simulink model "AD_SOAR_c7_V2f_c73_Clean_FullOrderControllerTest"  (R2022b)
settings: Solver=ode4  StartTime=0.0  StopTime=TMax  FixedStep=Control.DT  RelTol=1e-3
values from neighbouring files (symbols this model uses):
  dLPF_slow = c2d(ss(LPF_slow),Control.DT)    [C_BL_SOAR25_V2f_c73_Clean.m]    (also in C_BL_SOAR25_V2f_c73_Clean_original.m)
  DT = 0.0125    [hinf_controller.m]
  LPF_SetSmooth = Af_LPF(2*pi/10,1,Control.DT,1)    [C_BL_SOAR25_V2f_c73_Clean.m]    (also in C_BL_SOAR25_V2f_c73_Clean_original.m)
  OutList =     [OutList.mat]
  S_LowBPLim = 1    [C_BL_SOAR25_V2f_c73_Clean.m]    (also in C_BL_SOAR25_V2f_c73_Clean_original.m)
undefined symbols (not defined in the file or in its folder): Control, DiscIntNeverNeededParam, Downratelimiter, OLControlParams, Parameters, PitchControlParams, rpm2radps, Simulation, strmatch, TorqueControlParams, Upratelimiter
libraries: cstblocks x4, simulink x2, simulink_extras x1
settings Model: Creator=Hazim Namik  LastModifiedBy=aoifework
settings SolverCC: AlgebraicLoopSolver=LineSearch
settings DataIOCC: LimitDataPoints=on  SaveFormat=Array  ReturnWorkspaceOutputs=off  SignalLoggingName=sigsOut
settings OptimizationCC: BlockReduction=off  BooleanDataType=off  ReuseModelBlockBuffer=on  LifeSpan=inf
settings DebuggingCC: SaveWithParameterizedLinksMsg=none  UnderspecifiedInitializationDetection=Classic  MergeDetectMultiDrivingBlocksExec=none  UnconnectedInputMsg=warning  UnconnectedOutputMsg=warning  UnconnectedLineMsg=warning  AllowSymbolicDim=off  PregeneratedLibrarySubsystemCodeDiagnostic=none  SFUnexpectedBacktrackingDiag=warning  SFNoUnconditionalDefaultTransitionDiag=warning  SFExecutionAtInitializationDiag=none  ArithmeticOperatorsInVariantConditions=warning
settings HardwareCC: ProdBitPerPointer=32  ProdBitPerSizeT=32  ProdBitPerPtrDiffT=32  ProdLargestAtomicFloat=None  ProdIntDivRoundTo=Undefined  ProdEndianess=Unspecified  ProdWordSize=32  ProdHWDeviceType=32-bit Generic  TargetBitPerLong=64  TargetBitPerPointer=64  TargetBitPerSizeT=64  TargetBitPerPtrDiffT=64  TargetLongLongMode=on  TargetIntDivRoundTo=Zero  TargetEndianess=LittleEndian  TargetWordSize=64  TargetHWDeviceType=MATLAB Host  ProdEqTarget=off
settings ModelReferenceCC: EnableRefExpFcnMdlSchedulingChecks=on  PropagateSignalLabelsOutOfModel=off
settings SFSimCC: SimUseLocalCustomCode=off  CustomCodeUndefinedFunction=UseInterfaceOnly
settings RTWCC: RTWUseLocalCustomCode=off  DLArmComputeVersion=19.05
settings CodeAppCC: StateflowObjectComments=on
settings GRTTargetCC: TargetLangStandard=C89/C90 (ANSI)
settings ConfigComp: CovMetricSettings=dw  CovSaveCumulativeToWorkspaceVar=on  CovSaveSingleToWorkspaceVar=on  CovExternalEMLEnable=off  CovSFcnEnable=off

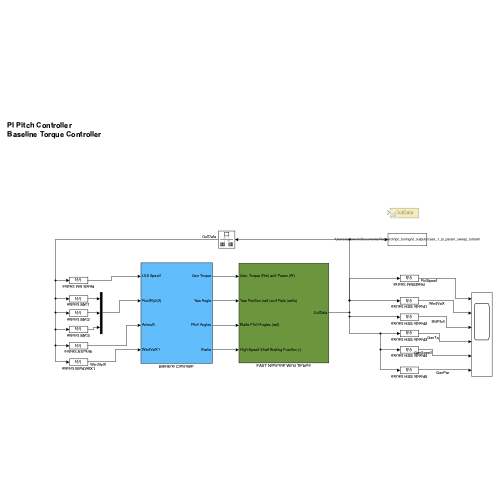
[thumbnail: Simulink's stored preview of the top-level diagram]
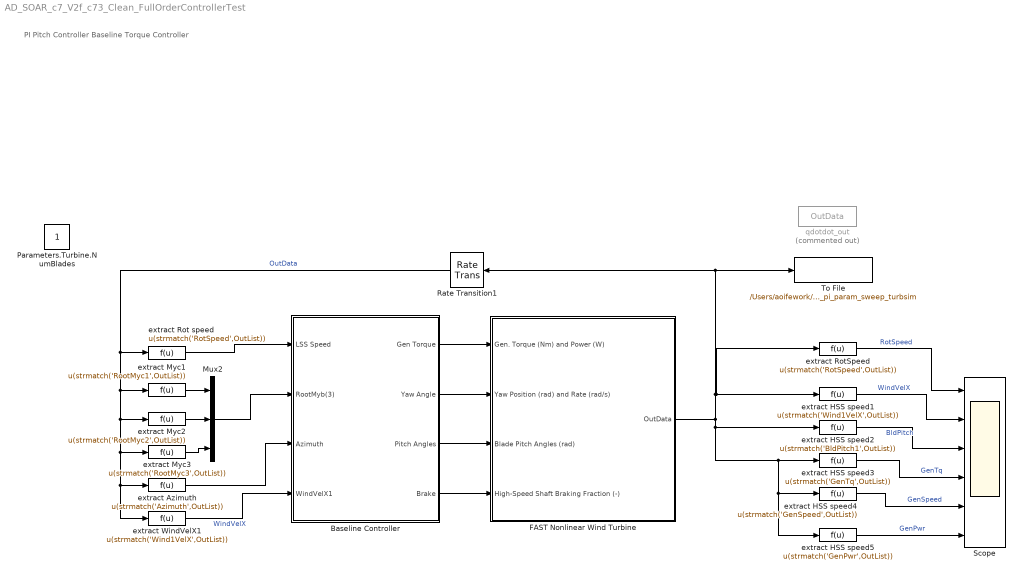
== system AD_SOAR_c7_V2f_c73_Clean_FullOrderControllerTest ==
  note: PI Pitch Controller
      | Baseline Torque Controller
  Baseline Controller : Subsystem
  FAST Nonlinear Wind Turbine : Subsystem  mask(FAST Nonlinear Wind Turbine){}
      mask help: This block contains the FAST S-Function.
      mask init:
      | clear FAST_SFunc
  Mux2 : Mux  Inputs=3
  Rate Transition1 : RateTransition
  Scope : Scope  NumInputPorts=6
  To File : ToFile  Filename=/Users/aoifework/Documents/Research/ipc_tuning/sl_outputs/case_1_pi_param_sweep_turbsim  MatrixName=OutData  SaveFormat=Timeseries
  extract Azimuth : Fcn  Expr=u(strmatch('Azimuth',OutList))
  extract HSS speed1 : Fcn  Expr=u(strmatch('Wind1VelX',OutList))
  extract HSS speed2 : Fcn  Expr=u(strmatch('BldPitch1',OutList))
  extract HSS speed3 : Fcn  Expr=u(strmatch('GenTq',OutList))
  extract HSS speed4 : Fcn  Expr=u(strmatch('GenSpeed',OutList))
  extract HSS speed5 : Fcn  Expr=u(strmatch('GenPwr',OutList))
  extract Myc1 : Fcn  Expr=u(strmatch('RootMyc1',OutList))
  extract Myc2 : Fcn  Expr=u(strmatch('RootMyc2',OutList))
  extract Myc3 : Fcn  Expr=u(strmatch('RootMyc3',OutList))
  extract Rot speed : Fcn  Expr=u(strmatch('RotSpeed',OutList))
  extract RotSpeed : Fcn  Expr=u(strmatch('RotSpeed',OutList))
  extract WindVelX1 : Fcn  Expr=u(strmatch('Wind1VelX',OutList))
  qdotdot_out : ToWorkspace  Commented=on  VariableName=OutData  SaveFormat=Structure With Time  SampleTime=-1
  Parameters.Turbine.NumBlades : Constant  IOType=siggen
  wires:
  Rate Transition1/1 -> extract Myc1/1, extract Myc2/1, extract Myc3/1, extract WindVelX1/1, extract Azimuth/1, extract Rot speed/1  "OutData"
  Baseline Controller/1(Gen Torque) -> FAST Nonlinear Wind Turbine/1(Gen. Torque (Nm) and Power (W))
  Baseline Controller/2(Yaw Angle) -> FAST Nonlinear Wind Turbine/2(Yaw Position (rad) and Rate (rad/s))
  Baseline Controller/3(Pitch Angles) -> FAST Nonlinear Wind Turbine/3(Blade Pitch Angles (rad))
  Baseline Controller/4(Brake) -> FAST Nonlinear Wind Turbine/4(High-Speed Shaft Braking Fraction (-))
  extract HSS speed1/1 -> Scope/2  "WindVelX"
  extract HSS speed2/1 -> Scope/3  "BldPitch"
  extract HSS speed3/1 -> Scope/4  "GenTq"
  extract HSS speed4/1 -> Scope/5  "GenSpeed"
  extract HSS speed5/1 -> Scope/6  "GenPwr"
  extract Rot speed/1 -> Baseline Controller/1(LSS Speed)
  FAST Nonlinear Wind Turbine/1(OutData) -> Rate Transition1/1, To File/1, extract RotSpeed/1, extract HSS speed1/1, extract HSS speed5/1, extract HSS speed4/1, extract HSS speed3/1, extract HSS speed2/1
  extract RotSpeed/1 -> Scope/1  "RotSpeed"
  extract Myc2/1 -> Mux2/2
  extract Azimuth/1 -> Baseline Controller/3(Azimuth)
  extract Myc1/1 -> Mux2/1
  extract Myc3/1 -> Mux2/3
  Mux2/1 -> Baseline Controller/2(RootMyb(3))
  extract WindVelX1/1 -> Baseline Controller/4(WindVelX1)  "WindVelX"

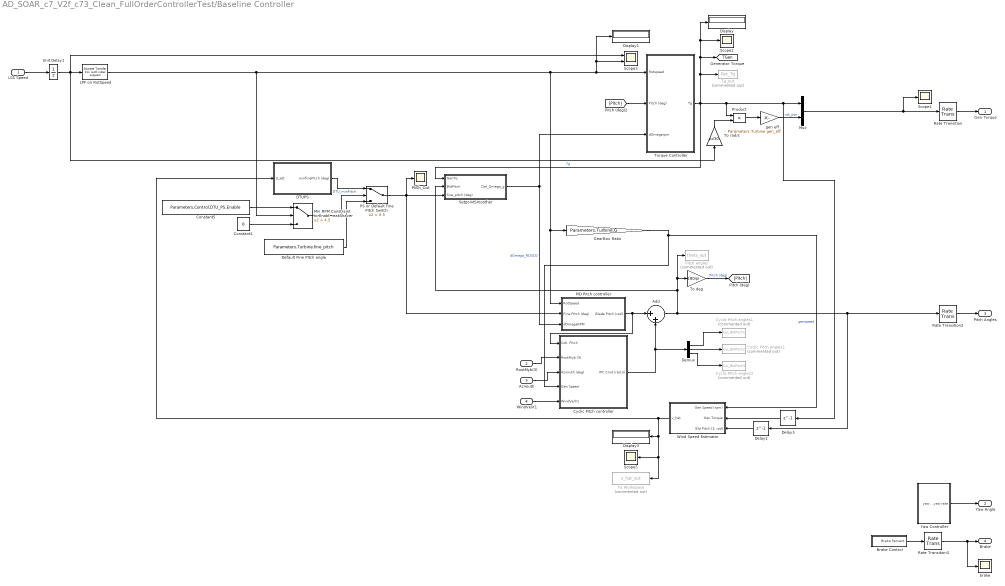
== system AD_SOAR_c7_V2f_c73_Clean_FullOrderControllerTest/Baseline Controller ==
  LSS Speed : Inport
  RootMyb(3) : Inport  Port=2
  Azimuth : Inport  Port=3
  WindVelX1 : Inport  Port=4
  Add : Sum  Inputs=|++
  Brake Control : Subsystem
  Constant1 : Constant  Value=0
  Constant5 : Constant  Value=Parameters.Control.DTU_PS.Enable
  Cyclic Pitch angles1 : ToWorkspace  Commented=on  VariableName=Cyc_BldPitch1  SampleTime=-1
  Cyclic Pitch angles2 : ToWorkspace  Commented=on  VariableName=Cyc_BldPitch2  SampleTime=-1
  Cyclic Pitch angles3 : ToWorkspace  Commented=on  VariableName=Cyc_BldPitch3  SampleTime=-1
  Cyclic Pitch controller : Subsystem  TreatAsAtomicUnit=on
      settings: MinAlgLoopOccurrences=on
  DTUPS : Subsystem
  Default Fine Pitch angle : Constant  Value=Parameters.Turbine.fine_pitch
  Delay2 : Delay  DelayLength=1  SampleTime=Control.DT
  Delay3 : Delay  DelayLength=1  SampleTime=Control.DT
  Demux : Demux  Outputs=3
  Display : Display
  Display1 : Display
  Display3 : Display
  GearBox Ratio : Gain  Gain=Parameters.Turbine.G
  LPF on RotSpeed : simulink_extras/Additional Discrete/Discrete Transfer Fcn (with initial outputs)  N=Parameters.LPF.LPnum  D=Parameters.LPF.LPden  U0=Parameters.Turbine.wr_min*Parameters.Turbine.G  Y0=Parameters.Turbine.wr_min*Parameters.Turbine.G  TS=Control.DT
  Min RPM Constraint to Enable PeakShaver : Switch  Criteria=u2 > Threshold  Threshold=4.5  SaturateOnIntegerOverflow=off  InputSameDT=off
  Mux : Mux  Inputs=2
  PID Pitch controller : Subsystem
      settings: MinAlgLoopOccurrences=on
  PS or Default Fine Pitch Switch : Switch  Criteria=u2 > Threshold  Threshold=0.5  SaturateOnIntegerOverflow=off  InputSameDT=off
  "Pitch angles " : ToWorkspace  Commented=on  VariableName=theta_out  SampleTime=-1
  PkSh_Out : Scope
  Product : Product  RndMeth=Zero
  Rate Transition : RateTransition  InitialCondition=[0,0]
  Rate Transition2 : RateTransition  InitialCondition=deg2rad(0)
  Rate Transition3 : RateTransition
  Scope1 : Scope
  Scope2 : Scope
  Scope3 : Scope  NumInputPorts=2
  Scope5 : Scope
  SetpointSmoother : Subsystem
  Tg_out : ToWorkspace  Commented=on  VariableName=Out_Tg  SampleTime=-1
      settings: MaxDataPoints=Inf
  To Workspace : ToWorkspace  Commented=on  VariableName=v_hat_out  SaveFormat=Timeseries  SampleTime=-1
  To deg : Gain  Gain=180/pi
  To rad/s : Gain  Gain=pi/30
  Torque Controller : Subsystem
  Unit Delay1 : UnitDelay  SampleTime=Control.DT  HasFrameUpgradeWarning=on
  Wind Speed Estimator : Subsystem
  Yaw Controller : Subsystem
  brake : Scope
  gen eff : Gain  Gain=Parameters.Turbine.gen_eff
  Gen Torque : Outport
  Yaw Angle : Outport  Port=2
  Pitch Angles : Outport  Port=3
  Brake : Outport  Port=4
  tag scope: TGen=global
  wires:
  Mux/1 -> Scope1/1, Rate Transition/1
  LSS Speed/1 -> Unit Delay1/1
  To deg/1 -> [Pitch]  "Pitch (deg)"
  Product/1 -> gen eff/1
  gen eff/1 -> Mux/2  "rot_pwr"
  [Pitch] -> Torque Controller/2(Pitch (deg))
  To rad/s/1 -> Product/2
  Unit Delay1/1 -> To rad/s/1, Scope3/1, LPF on RotSpeed/1
  Brake Control/1(Brake Percent) -> Rate Transition3/1
  Rate Transition/1 -> Gen Torque/1
  Yaw Controller/1(yaw and yaw rate) -> Yaw Angle/1
  Rate Transition2/1 -> Pitch Angles/1
  Rate Transition3/1 -> brake/1, Brake/1
  DTUPS/1(minfinePitch (deg)) -> PS or Default Fine Pitch Switch/1  "DTU_minPitch"
  Default Fine Pitch angle/1 -> PS or Default Fine Pitch Switch/3
  Wind Speed Estimator/1(v_hat) -> DTUPS/1(U_est), Display3/1, Scope5/1, To Workspace/1
  GearBox Ratio/1 -> Cyclic Pitch controller/4(Gen Speed), Wind Speed Estimator/1(Gen Speed (rpm))  "genspeed"
  LPF on RotSpeed/1 -> Min RPM Constraint to Enable PeakShaver/2, PID Pitch controller/1(RotSpeed), GearBox Ratio/1, Display1/1, Scope3/2, Torque Controller/1(Rotspeed)
  Torque Controller/1(Tg) -> SetpointSmoother/1(GenTq), Delay3/1, Mux/1, Product/1, Tg_out/1, [TGen], Display/1, Scope2/1  "Tg"
  SetpointSmoother/1(Del_Omega_g) -> PID Pitch controller/3(dOmegaRPM), Torque Controller/3(dOmegarpm)  "dOmega_ROSCO"
  Min RPM Constraint to Enable PeakShaver/1 -> PS or Default Fine Pitch Switch/2
  Constant5/1 -> Min RPM Constraint to Enable PeakShaver/1
  Constant1/1 -> Min RPM Constraint to Enable PeakShaver/3
  Delay2/1 -> Wind Speed Estimator/3("Bld Pitch (3, rad)")
  Delay3/1 -> Wind Speed Estimator/2(Gen Torque)
  RootMyb(3)/1 -> Cyclic Pitch controller/2(RootMyb (3))
  Azimuth/1 -> Cyclic Pitch controller/3(Azimuth (deg))
  Cyclic Pitch controller/1(IPC Cmd (rad,3)) -> Demux/1, Add/2
  PID Pitch controller/1(Blade Pitch (rad)) -> Cyclic Pitch controller/1(Coll. Pitch), Add/1
  PS or Default Fine Pitch Switch/1 -> SetpointSmoother/3(fine_pitch (deg)), PID Pitch controller/2(Fine Pitch (deg)), PkSh_Out/1
  Add/1 -> To deg/1, "Pitch angles "/1, SetpointSmoother/2(BldPitch), Rate Transition2/1, Delay2/1
  Demux/1 -> Cyclic Pitch angles1/1
  Demux/2 -> Cyclic Pitch angles2/1
  Demux/3 -> Cyclic Pitch angles3/1
  WindVelX1/1 -> Cyclic Pitch controller/5(WindVelX1)

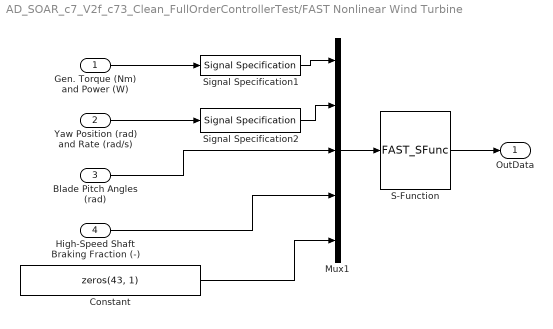
== system AD_SOAR_c7_V2f_c73_Clean_FullOrderControllerTest/FAST Nonlinear Wind Turbine ==
  Gen. Torque (Nm) and Power (W) : Inport
  Yaw Position (rad) and Rate (rad/s) : Inport  Port=2
  Blade Pitch Angles (rad) : Inport  Port=3
  High-Speed Shaft Braking Fraction (-) : Inport  Port=4
  Constant : Constant  Value=zeros(43, 1)
  Mux1 : Mux  Inputs=5
  S-Function : S-Function  FunctionName=FAST_SFunc  Parameters=FAST_InputFileName, TMax, 0  SFunctionDeploymentMode=off  EnableBusSupport=off
  Signal Specification1 : SignalSpecification  OutDataTypeStr=double  Dimensions=2
  Signal Specification2 : SignalSpecification  OutDataTypeStr=double  Dimensions=2
  OutData : Outport  VectorParamsAs1DForOutWhenUnconnected=off
  wires:
  Gen. Torque (Nm) and Power (W)/1 -> Signal Specification1/1
  S-Function/1 -> OutData/1
  Mux1/1 -> S-Function/1
  Blade Pitch Angles (rad)/1 -> Mux1/3
  Yaw Position (rad) and Rate (rad/s)/1 -> Signal Specification2/1
  Signal Specification1/1 -> Mux1/1
  Signal Specification2/1 -> Mux1/2
  High-Speed Shaft Braking Fraction (-)/1 -> Mux1/4
  Constant/1 -> Mux1/5

== system AD_SOAR_c7_V2f_c73_Clean_FullOrderControllerTest/Baseline Controller/Brake Control ==
  Brake : Constant  Value=Parameters.Turbine.Brake*100
  Brake Percent : Outport
  wires:
  Brake/1 -> Brake Percent/1

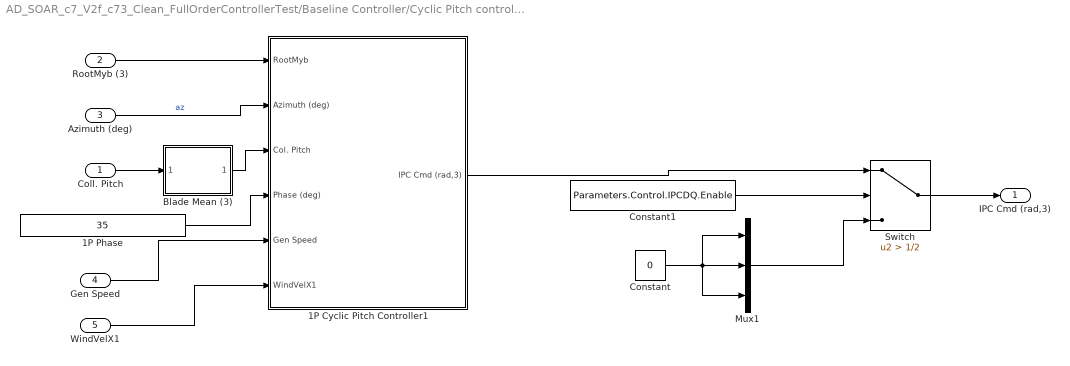
== system AD_SOAR_c7_V2f_c73_Clean_FullOrderControllerTest/Baseline Controller/Cyclic Pitch controller ==
  Coll. Pitch : Inport
  RootMyb (3) : Inport  Port=2
  Azimuth (deg) : Inport  Port=3
  Gen Speed : Inport  Port=4
  WindVelX1 : Inport  Port=5
  1P Cyclic Pitch Controller1 : Subsystem
  1P Phase : Constant  Value=35
  Blade Mean (3) : Subsystem
  Constant : Constant  Value=0
  Constant1 : Constant  Value=Parameters.Control.IPCDQ.Enable
  Mux1 : Mux  Inputs=3
  Switch : Switch  Criteria=u2 > Threshold  Threshold=1/2  SaturateOnIntegerOverflow=off  InputSameDT=off
  IPC Cmd (rad,3) : Outport  VectorParamsAs1DForOutWhenUnconnected=off
  wires:
  Azimuth (deg)/1 -> 1P Cyclic Pitch Controller1/2(Azimuth (deg))  "az"
  1P Phase/1 -> 1P Cyclic Pitch Controller1/4(Phase (deg))
  RootMyb (3)/1 -> 1P Cyclic Pitch Controller1/1(RootMyb)
  Blade Mean (3)/1(Output) -> 1P Cyclic Pitch Controller1/3(Col. Pitch)
  Coll. Pitch/1 -> Blade Mean (3)/1(Input (3))
  Gen Speed/1 -> 1P Cyclic Pitch Controller1/5(Gen Speed)
  Constant/1 -> Mux1/3, Mux1/1, Mux1/2
  Mux1/1 -> Switch/3
  Switch/1 -> IPC Cmd (rad,3)/1
  Constant1/1 -> Switch/2
  1P Cyclic Pitch Controller1/1(IPC Cmd (rad,3)) -> Switch/1
  WindVelX1/1 -> 1P Cyclic Pitch Controller1/6(WindVelX1)

== system AD_SOAR_c7_V2f_c73_Clean_FullOrderControllerTest/Baseline Controller/DTUPS ==
  U_est : Inport
  DTU PS Table : Lookup_n-D  NumberOfTableDimensions=1  BreakpointsForDimension1=Parameters.Control.DTU_PS.uu  Table=Parameters.Control.DTU_PS.pp  ExtrapMethod=Clip  InternalRulePriority=Speed  RndMeth=Simplest
  Discrete Filter1 : DiscreteFilter  Numerator=Parameters.Control.DTU_PS.TB_LPF.num{1}  Denominator=Parameters.Control.DTU_PS.TB_LPF.den{1}
  Saturation 0 to 90 deg5 : Saturate  UpperLimit=90  LowerLimit=Parameters.Turbine.fine_pitch
  Scope : Scope  NumInputPorts=2
  minfinePitch (deg) : Outport  VectorParamsAs1DForOutWhenUnconnected=off
  wires:
  DTU PS Table/1 -> Saturation 0 to 90 deg5/1, Scope/2
  U_est/1 -> Discrete Filter1/1
  Discrete Filter1/1 -> Scope/1, DTU PS Table/1  "DTU_MPu"
  Saturation 0 to 90 deg5/1 -> minfinePitch (deg)/1

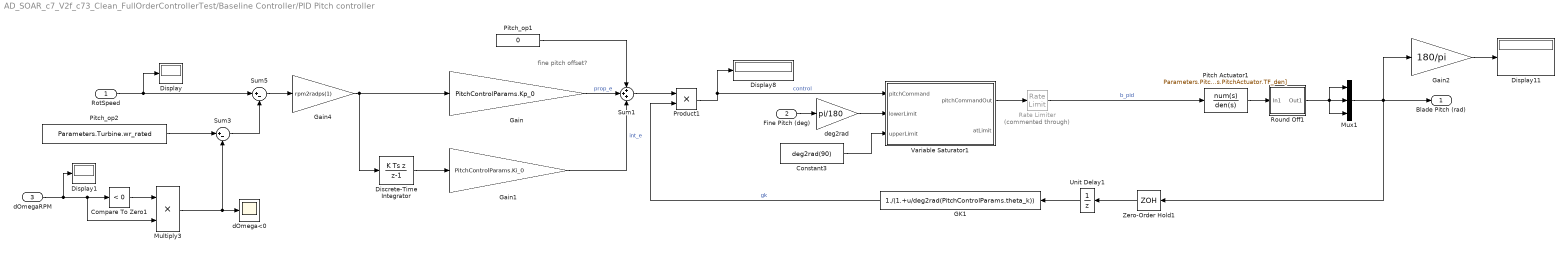
== system AD_SOAR_c7_V2f_c73_Clean_FullOrderControllerTest/Baseline Controller/PID Pitch controller ==
  note: fine pitch offset?
  RotSpeed : Inport
  Fine Pitch (deg) : Inport  Port=2
  dOmegaRPM : Inport  Port=3
  Compare To Zero1 : simulink/Logic and Bit Operations/Compare To Zero  relop=<  OutDataTypeStr=boolean
  Constant3 : Constant  Value=deg2rad(90)
  Discrete-Time Integrator : DiscreteIntegrator  IntegratorMethod=Integration: Backward Euler  gainval=1  InitialCondition=deg2rad(Parameters.Turbine.fine_pitch)/(PitchControlParams.Ki_0)/(1./(1.+deg2rad(Parameters.Turbine.fine_pitch)/PitchControlParams.theta_k))  SampleTime=Control.DT  LimitOutput=on  UpperSaturationLimit=5*1.570796/(PitchControlParams.Ki_0)/(1./(1.+1.570796/PitchControlParams.theta_k))  LowerSaturationLimit=deg2rad(Parameters.Turbine.fine_pitch)/(PitchControlParams.Ki_0)/(1./(1.+deg2rad(Parameters.Turbine.fine_pitch)/PitchControlParams.theta_k))  ICPrevOutput=DiscIntNeverNeededParam  ICPrevScaledInput=DiscIntNeverNeededParam
  Display{,1,8,11} (4 alike) : Display
  GK1 : Fcn  Expr=1./(1.+u/deg2rad(PitchControlParams.theta_k))
  Gain : Gain  Gain=PitchControlParams.Kp_0
  Gain1 : Gain  Gain=PitchControlParams.Ki_0
  Gain2 : Gain  Gain=180/pi
  Gain4 : Gain  Gain=rpm2radps(1)
  Multiply3 : Product
  Mux1 : Mux  Inputs=3
  Pitch Actuator1 : TransferFcn  Numerator=Parameters.PitchActuator.TF_num  Denominator=[Parameters.PitchActuator.TF_den]
  Pitch_op1 : Constant  Value=0  SampleTime=Control.DT
  Pitch_op2 : Constant  Value=Parameters.Turbine.wr_rated  SampleTime=Control.DT
  Product1 : Product  RndMeth=Zero
  Rate Limiter : RateLimiter  Commented=through  RisingSlewLimit=2.5*pi/180  FallingSlewLimit=- 2.5*pi/180  SampleTimeMode=inherited  InitialCondition=deg2rad(0)
  Round Off1 : Subsystem
  Sum1 : Sum  Inputs=+++
  Sum3 : Sum  Inputs=|+-  InputSameDT=on  SaturateOnIntegerOverflow=on  OutDataTypeStr=Inherit: Same as first input
  Sum5 : Sum  Inputs=|+-  InputSameDT=on  SaturateOnIntegerOverflow=on  OutDataTypeStr=Inherit: Same as first input
  Unit Delay1 : UnitDelay  InitialCondition=Parameters.Turbine.IC.Wg  SampleTime=Control.DT  HasFrameUpgradeWarning=on
  Variable Saturator1 : MATLAB Function  TreatAsAtomicUnit=on
  Zero-Order Hold1 : ZeroOrderHold  SampleTime=Control.DT
  dOmega<0 : Scope
  deg2rad : Gain  Gain=pi/180
  Blade Pitch (rad) : Outport
  wires:
  Zero-Order Hold1/1 -> Unit Delay1/1
  Rate Limiter/1 -> Pitch Actuator1/1  "b_pid"
  Pitch Actuator1/1 -> Round Off1/1(In1)
  Unit Delay1/1 -> GK1/1
  Variable Saturator1/1(pitchCommandOut) -> Rate Limiter/1
  Gain/1 -> Sum1/2  "prop_e"
  Gain1/1 -> Sum1/3  "int_e"
  Discrete-Time Integrator/1 -> Gain1/1
  RotSpeed/1 -> Display/1, Sum5/1
  Pitch_op1/1 -> Sum1/1
  Gain4/1 -> Gain/1, Discrete-Time Integrator/1
  Sum5/1 -> Gain4/1
  Sum1/1 -> Product1/1
  Round Off1/1(Out1) -> Mux1/3, Mux1/1, Mux1/2
  Product1/1 -> Variable Saturator1/1(pitchCommand), Display8/1  "control"
  GK1/1 -> Product1/2  "gk"
  Mux1/1 -> Gain2/1, Blade Pitch (rad)/1, Zero-Order Hold1/1
  Gain2/1 -> Display11/1
  deg2rad/1 -> Variable Saturator1/2(lowerLimit)
  Constant3/1 -> Variable Saturator1/3(upperLimit)
  Fine Pitch (deg)/1 -> deg2rad/1
  Multiply3/1 -> dOmega<0/1, Sum3/2
  dOmegaRPM/1 -> Display1/1, Compare To Zero1/1, Multiply3/2
  Compare To Zero1/1 -> Multiply3/1
  Pitch_op2/1 -> Sum3/1
  Sum3/1 -> Sum5/2

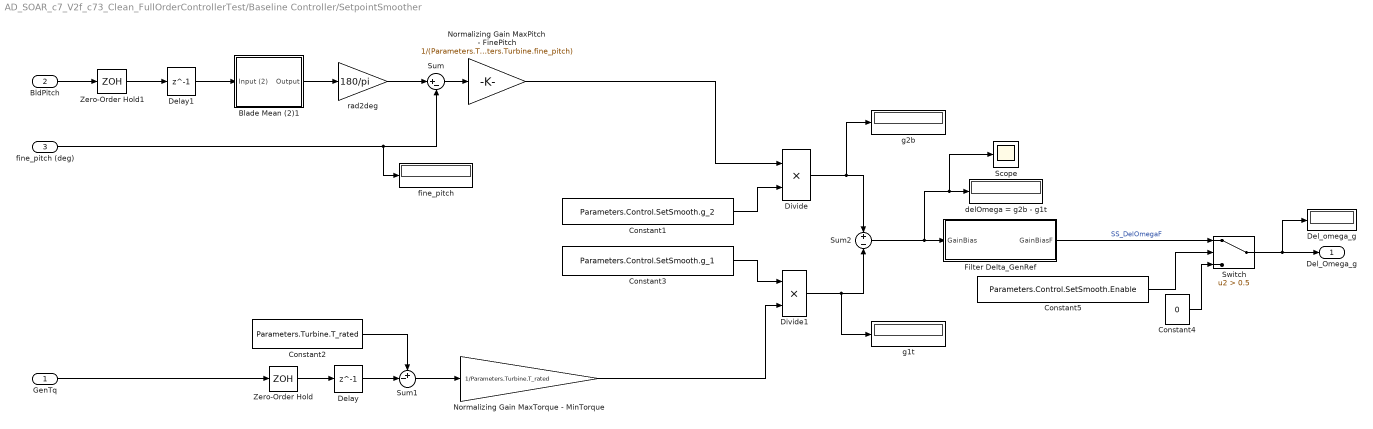
== system AD_SOAR_c7_V2f_c73_Clean_FullOrderControllerTest/Baseline Controller/SetpointSmoother ==
  GenTq : Inport
  BldPitch : Inport  Port=2
  fine_pitch (deg) : Inport  Port=3
  Blade Mean (2)1 : Subsystem
  Constant1 : Constant  Value=Parameters.Control.SetSmooth.g_2
  Constant2 : Constant  Value=Parameters.Turbine.T_rated
  Constant3 : Constant  Value=Parameters.Control.SetSmooth.g_1
  Constant4 : Constant  Value=0
  Constant5 : Constant  Value=Parameters.Control.SetSmooth.Enable
  Del_omega_g : Display
  Delay : Delay  DelayLength=1  InitialCondition=Parameters.Turbine.T_rated
  Delay1 : Delay  DelayLength=1  InitialCondition=Parameters.Turbine.fine_pitch
  Divide : Product  Inputs=**
  Divide1 : Product  Inputs=**
  Filter Delta_GenRef : Subsystem
  Normalizing Gain MaxPitch - FinePitch : Gain  Gain=1/(Parameters.Turbine.max_pitch - Parameters.Turbine.fine_pitch)
  Normalizing Gain MaxTorque - MinTorque : Gain  Gain=1/Parameters.Turbine.T_rated
  Scope : Scope
  Sum : Sum  Inputs=|+-
  Sum1 : Sum  Inputs=+-|
  Sum2 : Sum  Inputs=+|-
  Switch : Switch  Criteria=u2 > Threshold  Threshold=0.5  SaturateOnIntegerOverflow=off  InputSameDT=off
  Zero-Order Hold : ZeroOrderHold  SampleTime=Control.DT
  Zero-Order Hold1 : ZeroOrderHold  SampleTime=Control.DT
  delOmega = g2b - g1t : Display
  fine_pitch : Display
  g1t : Display
  g2b : Display
  rad2deg : Gain  Gain=180/pi
  Del_Omega_g : Outport  VectorParamsAs1DForOutWhenUnconnected=off
  wires:
  Divide1/1 -> g1t/1, Sum2/2
  Divide/1 -> g2b/1, Sum2/1
  Constant3/1 -> Divide1/1
  Constant1/1 -> Divide/2
  Sum/1 -> Normalizing Gain MaxPitch - FinePitch/1
  Sum2/1 -> Scope/1, delOmega = g2b - g1t/1, Filter Delta_GenRef/1(GainBias)
  Constant2/1 -> Sum1/1
  Sum1/1 -> Normalizing Gain MaxTorque - MinTorque/1
  Normalizing Gain MaxPitch - FinePitch/1 -> Divide/1
  Normalizing Gain MaxTorque - MinTorque/1 -> Divide1/2
  Filter Delta_GenRef/1(GainBiasF) -> Switch/1  "SS_DelOmegaF"
  rad2deg/1 -> Sum/1
  fine_pitch (deg)/1 -> fine_pitch/1, Sum/2
  Zero-Order Hold1/1 -> Delay1/1
  Delay1/1 -> Blade Mean (2)1/1(Input (2))
  BldPitch/1 -> Zero-Order Hold1/1
  Blade Mean (2)1/1(Output) -> rad2deg/1
  Zero-Order Hold/1 -> Delay/1
  GenTq/1 -> Zero-Order Hold/1
  Delay/1 -> Sum1/2
  Switch/1 -> Del_omega_g/1, Del_Omega_g/1
  Constant4/1 -> Switch/3
  Constant5/1 -> Switch/2

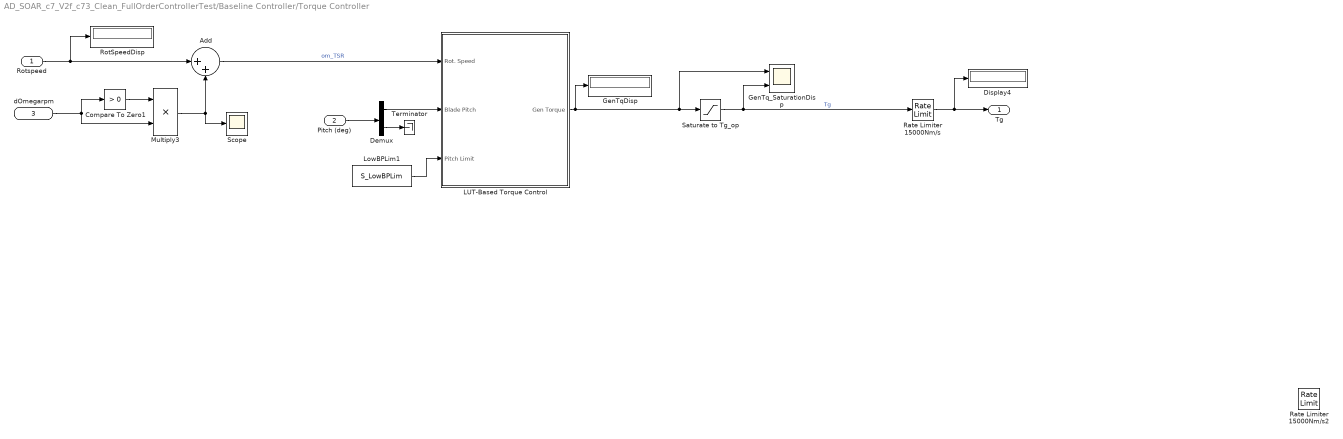
== system AD_SOAR_c7_V2f_c73_Clean_FullOrderControllerTest/Baseline Controller/Torque Controller ==
  Rotspeed : Inport
  Pitch (deg) : Inport  Port=2
  dOmegarpm : Inport  Port=3
  Add : Sum  Inputs=|++
  Compare To Zero1 : simulink/Logic and Bit Operations/Compare To Zero  relop=>  OutDataTypeStr=boolean
  Demux : Demux  Outputs=[1, 2]
  Display4 : Display
  GenTqDisp : Display
  GenTq_SaturationDisp : Scope  NumInputPorts=2
  LUT-Based Torque Control : Subsystem
  LowBPLim1 : Constant  Value=S_LowBPLim  SampleTime=Control.DT
  Multiply3 : Product
  Rate Limiter 15000Nm/s : RateLimiter  RisingSlewLimit=Upratelimiter.Disable  FallingSlewLimit=Downratelimiter.Disable  SampleTimeMode=inherited
  Rate Limiter 15000Nm/s2 : RateLimiter  RisingSlewLimit=51922763.3  FallingSlewLimit=- 500000  SampleTimeMode=inherited
  RotSpeedDisp : Display
  Saturate to Tg_op : Saturate  UpperLimit=TorqueControlParams.T_rated  LowerLimit=0
  Scope : Scope
  Terminator : Terminator
  Tg : Outport
  wires:
  Rotspeed/1 -> Add/1, RotSpeedDisp/1
  Pitch (deg)/1 -> Demux/1
  Demux/1 -> LUT-Based Torque Control/2(Blade Pitch)
  Demux/2 -> Terminator/1
  LowBPLim1/1 -> LUT-Based Torque Control/3(Pitch Limit)
  Saturate to Tg_op/1 -> Rate Limiter 15000Nm/s/1, GenTq_SaturationDisp/2  "Tg"
  LUT-Based Torque Control/1(Gen Torque) -> Saturate to Tg_op/1, GenTq_SaturationDisp/1, GenTqDisp/1
  Rate Limiter 15000Nm/s/1 -> Display4/1, Tg/1
  Compare To Zero1/1 -> Multiply3/1
  dOmegarpm/1 -> Compare To Zero1/1, Multiply3/2
  Multiply3/1 -> Add/2, Scope/1
  Add/1 -> LUT-Based Torque Control/1(Rot. Speed)  "om_TSR"

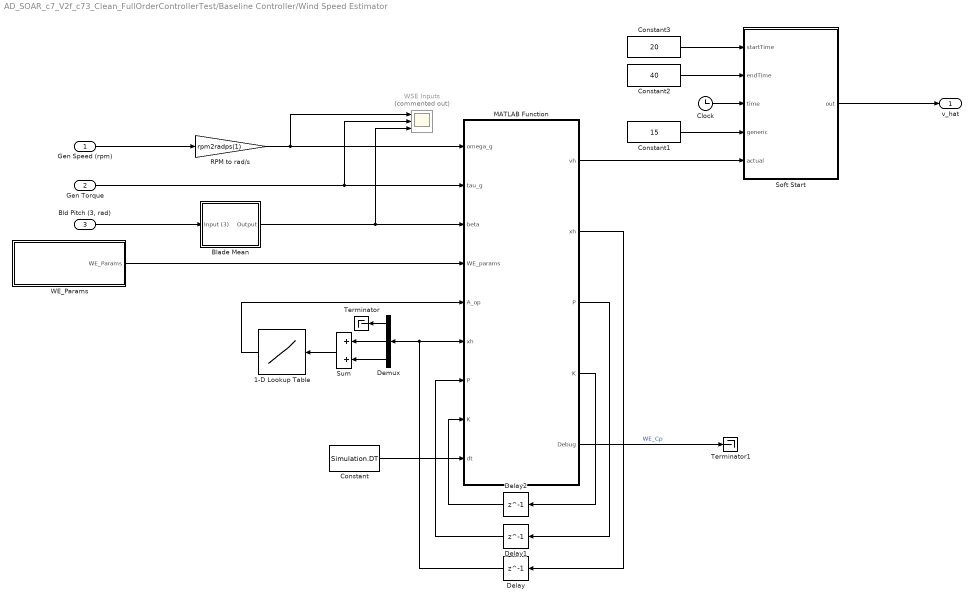
== system AD_SOAR_c7_V2f_c73_Clean_FullOrderControllerTest/Baseline Controller/Wind Speed Estimator ==
  Gen Speed (rpm) : Inport
  Gen Torque : Inport  Port=2
  "Bld Pitch (3, rad)" : Inport  Port=3
  1-D Lookup Table : Lookup_n-D  NumberOfTableDimensions=1  BreakpointsForDimension1=[-5:5]  Table=tanh([-5:5])  InternalRulePriority=Speed  RndMeth=Simplest
  "Blade Mean " : Subsystem
  Clock : Clock
  Constant : Constant  Value=Simulation.DT
  Constant1 : Constant  Value=15
  Constant2 : Constant  Value=40
  Constant3 : Constant  Value=20
  Delay : Delay  DelayLength=1  InitialCondition=[Parameters.Turbine.G, 0, Parameters.Control.WSE.v0]'
  Delay1 : Delay  DelayLength=1  InitialCondition=diag([0.1, 0.1, 1])^2
  Delay2 : Delay  DelayLength=1  InitialCondition=zeros(3,1)
  Demux : Demux  Outputs=3
  MATLAB Function : MATLAB Function  TreatAsAtomicUnit=on
  RPM to rad/s : Gain  Gain=rpm2radps(1)
  Soft Start : MATLAB Function  TreatAsAtomicUnit=on
  Sum : Sum
  Terminator : Terminator
  Terminator1 : Terminator
  WE_Params : Subsystem
  WSE Inputs : Scope  Commented=on  NumInputPorts=3
  v_hat : Outport  VectorParamsAs1DForOutWhenUnconnected=off
  wires:
  MATLAB Function/2(xh) -> Delay/1
  Delay/1 -> Demux/1, MATLAB Function/6("xh ")
  MATLAB Function/3(P) -> Delay1/1
  Delay1/1 -> MATLAB Function/7("P ")
  Gen Torque/1 -> MATLAB Function/2(tau_g), WSE Inputs/2
  MATLAB Function/4(K) -> Delay2/1
  Delay2/1 -> MATLAB Function/8("K ")
  Constant/1 -> MATLAB Function/9(dt)
  Demux/2 -> Sum/1
  Demux/3 -> Sum/2
  Demux/1 -> Terminator/1
  Sum/1 -> 1-D Lookup Table/1
  1-D Lookup Table/1 -> MATLAB Function/5(A_op)
  WE_Params/1(WE_Params) -> MATLAB Function/4(WE_params)
  Clock/1 -> Soft Start/3(time)
  Constant1/1 -> Soft Start/4(generic)
  Constant2/1 -> Soft Start/2(endTime)
  Constant3/1 -> Soft Start/1(startTime)
  MATLAB Function/1(vh) -> Soft Start/5(actual)
  Soft Start/1(out) -> v_hat/1
  MATLAB Function/5(Debug) -> Terminator1/1  "WE_Cp"
  "Bld Pitch (3, rad)"/1 -> "Blade Mean "/1(Input (3))
  "Blade Mean "/1(Output) -> WSE Inputs/3, MATLAB Function/3(beta)
  Gen Speed (rpm)/1 -> RPM to rad/s/1
  RPM to rad/s/1 -> WSE Inputs/1, MATLAB Function/1(omega_g)

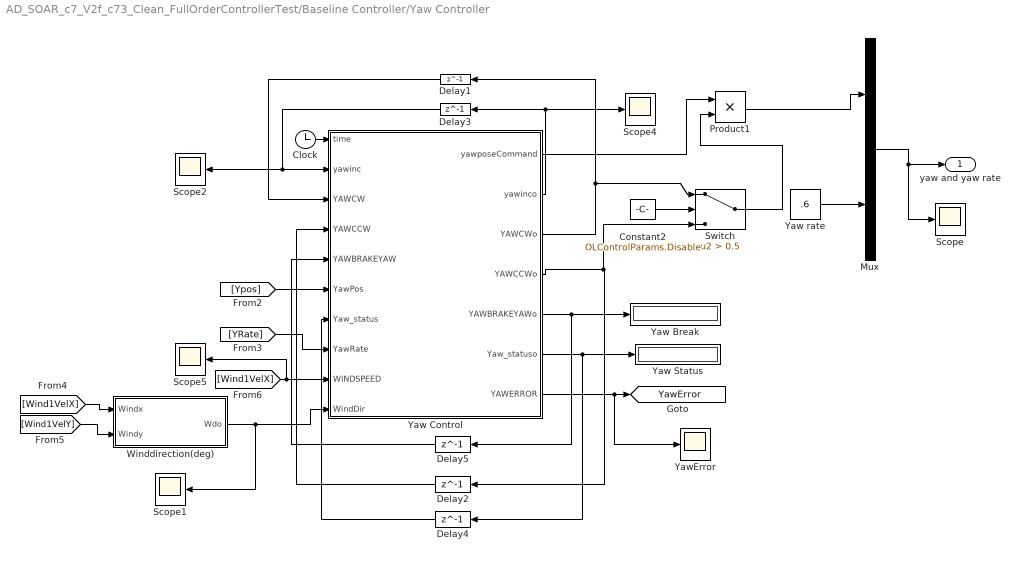
== system AD_SOAR_c7_V2f_c73_Clean_FullOrderControllerTest/Baseline Controller/Yaw Controller ==
  " Yaw Control" : MATLAB Function  TreatAsAtomicUnit=on
  Clock : Clock
  Constant2 : Constant  Value=OLControlParams.Disable
  Delay{1..5} (5 alike) : Delay  DelayLength=1  InitialCondition=0
  Mux : Mux  Inputs=2
  Product1 : Product
  Scope{,1..2,4..5} (5 alike) : Scope
  Switch : Switch  Criteria=u2 > Threshold  Threshold=0.5  SaturateOnIntegerOverflow=off  InputSameDT=off
  Winddirection(deg) : MATLAB Function  TreatAsAtomicUnit=on
  Yaw Break : Display
      settings: Decimation=2
  Yaw Status : Display
      settings: Decimation=2
  Yaw rate : Constant  Value=.6
  YawError : Scope
  yaw and yaw rate : Outport
  tag scope: YawError=global
  wires:
  Mux/1 -> Scope/1, yaw and yaw rate/1
  ? -> ?
  Clock/1 -> " Yaw Control"/1(time)
  [Ypos] -> " Yaw Control"/6(YawPos)
  [YRate] -> " Yaw Control"/8(YawRate)
  " Yaw Control"/2(yawinco) -> Scope4/1, Delay3/1
  Yaw rate/1 -> Mux/2
  Delay4/1 -> " Yaw Control"/7(Yaw_status)
  [Wind1VelY] -> Winddirection(deg)/2(Windy)
  [Wind1VelX] -> Winddirection(deg)/1(Windx)
  Winddirection(deg)/1(Wdo) -> " Yaw Control"/10(WindDir), Scope1/1
  " Yaw Control"/6(Yaw_statuso) -> Delay4/1, Yaw Status/1
  " Yaw Control"/3(YAWCWo) -> Switch/1, Delay1/1
  Delay1/1 -> " Yaw Control"/3(YAWCW)
  [Wind1VelX] -> " Yaw Control"/9(WINDSPEED), Scope5/1
  " Yaw Control"/1(yawposeCommand) -> Product1/1
  " Yaw Control"/4(YAWCCWo) -> Switch/3, Delay2/1
  Delay2/1 -> " Yaw Control"/4(YAWCCW)
  Delay3/1 -> " Yaw Control"/2(yawinc), Scope2/1
  Switch/1 -> Product1/2
  Product1/1 -> Mux/1
  " Yaw Control"/5(YAWBRAKEYAWo) -> Delay5/1, Yaw Break/1
  Delay5/1 -> " Yaw Control"/5(YAWBRAKEYAW)
  " Yaw Control"/7(YAWERROR) -> YawError/1, [YawError]
  Constant2/1 -> Switch/2

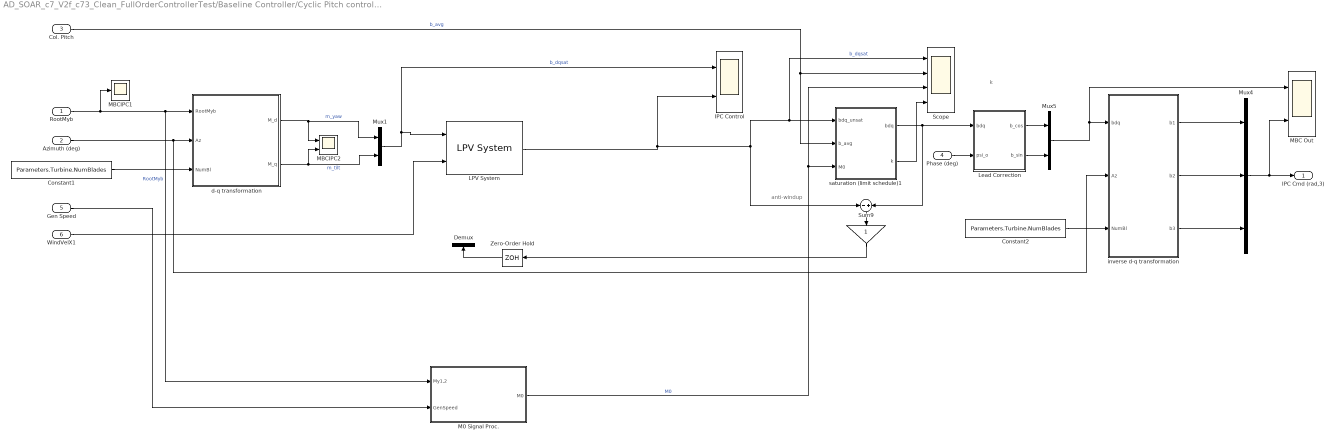
== system AD_SOAR_c7_V2f_c73_Clean_FullOrderControllerTest/Baseline Controller/Cyclic Pitch controller/1P Cyclic Pitch Controller1 ==
  note: k
  note: anti-windup
  RootMyb : Inport
  Azimuth (deg) : Inport  Port=2
  Col. Pitch : Inport  Port=3
  Phase (deg) : Inport  Port=4
  Gen Speed : Inport  Port=5
  WindVelX1 : Inport  Port=6
  " " : Gain
  Constant1 : Constant  Value=Parameters.Turbine.NumBlades
  Constant2 : Constant  Value=Parameters.Turbine.NumBlades
  Demux : Demux  Outputs=2
  IPC Control : Scope  NumInputPorts=2
  LPV System : cstblocks/Linear Parameter Varying/LPV System  sys=K_IPC  x0=0  uOffset=0  yOffset=0  xOffset=0  opEquilOption=on  dxOffset=0  sysFixedOption=Use the first model in state-space array  sysFixed=[]  AFixed=false  BFixed=false  CFixed=false  DFixed=false  uDelayFixed=false  yDelayFixed=false  iDelayFixed=false  IMethod=Linear  EMethod=Clip  IndexSearch=Binary search  IndexBegin=on  OutputX=off  OutputXdot=off  OutputLTI=off  OutputOP=off  DataType=double  SimMode=Interpreted execution  InitBufferSize=1024  FixedBuffer=off
  Lead Correction : MATLAB Function  TreatAsAtomicUnit=on
  M0 Signal Proc. : Subsystem
  MBC Out : Scope  NumInputPorts=2
  MBCIPC1 : Scope
  MBCIPC2 : Scope  NumInputPorts=2
  Mux1 : Mux  Inputs=2
  Mux4 : Mux  Inputs=3
  Mux5 : Mux  Inputs=2
  Scope : Scope  NumInputPorts=4
  Sum9 : Sum  Inputs=-|+
  Zero-Order Hold : ZeroOrderHold  SampleTime=DT
  d-q transformation : MATLAB Function  TreatAsAtomicUnit=on
  inverse d-q transformation : MATLAB Function  TreatAsAtomicUnit=on
  saturation (limit schedule)1 : MATLAB Function  TreatAsAtomicUnit=on
  IPC Cmd (rad,3) : Outport  VectorParamsAs1DForOutWhenUnconnected=off
  wires:
  M0 Signal Proc./1(M0) -> saturation (limit schedule)1/3(M0), Scope/3  "M0"
  Col. Pitch/1 -> Scope/2, saturation (limit schedule)1/2(b_avg)  "b_avg"
  saturation (limit schedule)1/1(bdq) -> Lead Correction/1(bdq), Sum9/2
  Gen Speed/1 -> M0 Signal Proc./2(GenSpeed)
  d-q transformation/1(M_d) -> Mux1/1, MBCIPC2/1  "m_yaw"
  Mux5/1 -> inverse d-q transformation/1(bdq), MBC Out/1
  inverse d-q transformation/3(b3) -> Mux4/3
  Phase (deg)/1 -> Lead Correction/2(psi_o)
  inverse d-q transformation/1(b1) -> Mux4/1
  inverse d-q transformation/2(b2) -> Mux4/2
  Mux4/1 -> IPC Cmd (rad,3)/1, MBC Out/2
  Zero-Order Hold/1 -> Demux/1
  " "/1 -> Zero-Order Hold/1
  LPV System/1 -> IPC Control/2, Sum9/1, saturation (limit schedule)1/1(bdq_unsat), Scope/1  "b_dqsat"
  RootMyb/1 -> M0 Signal Proc./1(My1,2), d-q transformation/1(RootMyb), MBCIPC1/1  "RootMyb"
  Sum9/1 -> " "/1
  Azimuth (deg)/1 -> inverse d-q transformation/2(Az), d-q transformation/2(Az)
  Lead Correction/1(b_cos) -> Mux5/1
  Lead Correction/2(b_sin) -> Mux5/2
  saturation (limit schedule)1/2(k) -> Scope/4
  Constant1/1 -> d-q transformation/3(NumBl)
  Constant2/1 -> inverse d-q transformation/3(NumBl)
  d-q transformation/2(M_q) -> Mux1/2, MBCIPC2/2  "m_tilt"
  Mux1/1 -> LPV System/1, IPC Control/1  "b_dqsat"
  WindVelX1/1 -> LPV System/2

== system AD_SOAR_c7_V2f_c73_Clean_FullOrderControllerTest/Baseline Controller/Cyclic Pitch controller/Blade Mean (3) ==
  Input (3) : Inport
  Add : Sum  Inputs=+++
  Demux : Demux  Outputs=3
  Gain : Gain  Gain=1/Parameters.Turbine.NumBlades
  Output : Outport  VectorParamsAs1DForOutWhenUnconnected=off
  wires:
  Input (3)/1 -> Demux/1
  Gain/1 -> Output/1
  Demux/1 -> Add/1
  Demux/2 -> Add/2
  Add/1 -> Gain/1
  Demux/3 -> Add/3

== system AD_SOAR_c7_V2f_c73_Clean_FullOrderControllerTest/Baseline Controller/PID Pitch controller/Round Off1 ==
  In1 : Inport
  Gain2 : Gain  Gain=1e10
  Gain3 : Gain  Gain=1e-10
  Rounding Function : Rounding  Operator=round
  Out1 : Outport
  wires:
  In1/1 -> Gain2/1
  Gain3/1 -> Out1/1
  Rounding Function/1 -> Gain3/1
  Gain2/1 -> Rounding Function/1

== system AD_SOAR_c7_V2f_c73_Clean_FullOrderControllerTest/Baseline Controller/SetpointSmoother/Blade Mean (2)1 ==
  Input (2) : Inport
  Add : Sum  Inputs=+++
  Demux : Demux  Outputs=3
  Gain : Gain  Gain=1/Parameters.Turbine.NumBlades
  Output : Outport  VectorParamsAs1DForOutWhenUnconnected=off
  wires:
  Input (2)/1 -> Demux/1
  Gain/1 -> Output/1
  Demux/1 -> Add/1
  Demux/2 -> Add/2
  Add/1 -> Gain/1
  Demux/3 -> Add/3

== system AD_SOAR_c7_V2f_c73_Clean_FullOrderControllerTest/Baseline Controller/SetpointSmoother/Filter Delta_GenRef ==
  GainBias : Inport
  Discrete Filter : DiscreteFilter  Numerator=LPF_SetSmooth.num{1}  Denominator=LPF_SetSmooth.den{1}  SampleTime=Control.DT
  GainBiasF : Outport  VectorParamsAs1DForOutWhenUnconnected=off
  wires:
  Discrete Filter/1 -> GainBiasF/1
  GainBias/1 -> Discrete Filter/1

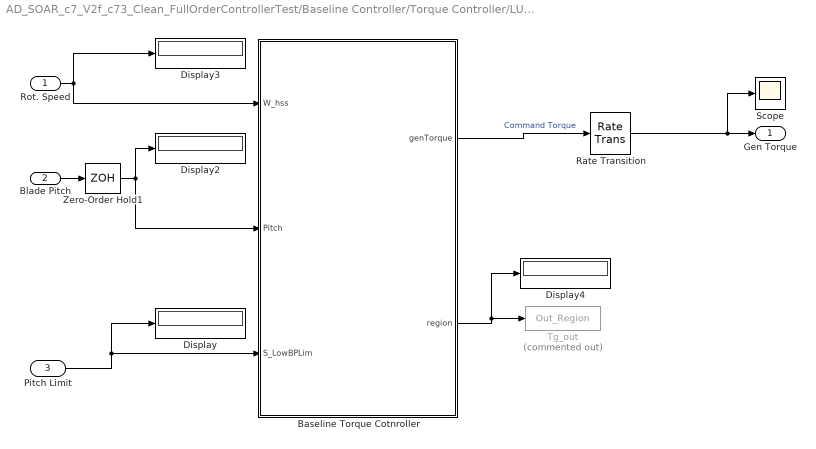
== system AD_SOAR_c7_V2f_c73_Clean_FullOrderControllerTest/Baseline Controller/Torque Controller/LUT-Based Torque Control ==
  Rot. Speed : Inport
  Blade Pitch : Inport  Port=2
  Pitch Limit : Inport  Port=3
  Baseline Torque Cotnroller : MATLAB Function  TreatAsAtomicUnit=on
  Display{,2..4} (4 alike) : Display
  Rate Transition : RateTransition
  Scope : Scope
  Tg_out : ToWorkspace  Commented=on  VariableName=Out_Region  SampleTime=-1
      settings: MaxDataPoints=Inf
  Zero-Order Hold1 : ZeroOrderHold  SampleTime=Control.DT
  Gen Torque : Outport
  wires:
  Baseline Torque Cotnroller/1(genTorque) -> Rate Transition/1  "Command Torque"
  Baseline Torque Cotnroller/2(region) -> Display4/1, Tg_out/1
  Blade Pitch/1 -> Zero-Order Hold1/1
  Pitch Limit/1 -> Baseline Torque Cotnroller/3(S_LowBPLim), Display/1
  Rate Transition/1 -> Scope/1, Gen Torque/1
  Zero-Order Hold1/1 -> Baseline Torque Cotnroller/2(Pitch), Display2/1
  Rot. Speed/1 -> Baseline Torque Cotnroller/1(W_hss), Display3/1

== system AD_SOAR_c7_V2f_c73_Clean_FullOrderControllerTest/Baseline Controller/Wind Speed Estimator/Blade Mean  ==
  Input (3) : Inport
  Add : Sum  Inputs=+++
  Demux : Demux  Outputs=3
  Gain : Gain  Gain=1/Parameters.Turbine.NumBlades
  Output : Outport  VectorParamsAs1DForOutWhenUnconnected=off
  wires:
  Input (3)/1 -> Demux/1
  Gain/1 -> Output/1
  Demux/1 -> Add/1
  Demux/2 -> Add/2
  Add/1 -> Gain/1
  Demux/3 -> Add/3

== system AD_SOAR_c7_V2f_c73_Clean_FullOrderControllerTest/Baseline Controller/Wind Speed Estimator/WE_Params ==
  Constant1 : Constant  Value=Parameters.Turbine.Jtot
  Constant2 : Constant  Value=Parameters.Turbine.rho
  Constant3 : Constant  Value=Parameters.Turbine.R
  Constant4 : Constant  Value=Parameters.Turbine.G
  Constant5 : Constant  Value=Parameters.Turbine.ConeAngle
  Constant6 : Constant  Value=Parameters.Turbine.ShaftTilt
  Mux : Mux  Inputs=6
  WE_Params : Outport
  wires:
  Constant2/1 -> Mux/2
  Mux/1 -> WE_Params/1
  Constant4/1 -> Mux/4
  Constant1/1 -> Mux/1
  Constant3/1 -> Mux/3
  Constant5/1 -> Mux/5
  Constant6/1 -> Mux/6

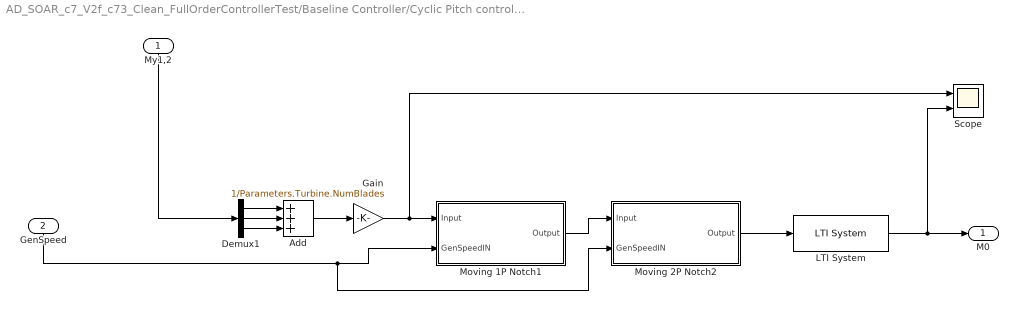
== system AD_SOAR_c7_V2f_c73_Clean_FullOrderControllerTest/Baseline Controller/Cyclic Pitch controller/1P Cyclic Pitch Controller1/M0 Signal Proc. ==
  My1,2 : Inport
  GenSpeed : Inport  Port=2
  Add : Sum  Inputs=+++
  Demux1 : Demux  Outputs=3
  Gain : Gain  Gain=1/Parameters.Turbine.NumBlades
  LTI System : cstblocks/LTI System  sys=LSM0_LPF  IC=[]
  Moving 1P Notch1 : Subsystem
  Moving 2P Notch2 : Subsystem
  Scope : Scope  NumInputPorts=2
  M0 : Outport  VectorParamsAs1DForOutWhenUnconnected=off
  wires:
  Gain/1 -> Moving 1P Notch1/1(Input), Scope/1
  Moving 1P Notch1/1(Output) -> Moving 2P Notch2/1(Input)
  Demux1/1 -> Add/1
  Demux1/2 -> Add/2
  Add/1 -> Gain/1
  Moving 2P Notch2/1(Output) -> LTI System/1
  My1,2/1 -> Demux1/1
  GenSpeed/1 -> Moving 1P Notch1/2(GenSpeedIN), Moving 2P Notch2/2(GenSpeedIN)
  LTI System/1 -> M0/1, Scope/2
  Demux1/3 -> Add/3

== system AD_SOAR_c7_V2f_c73_Clean_FullOrderControllerTest/Baseline Controller/Cyclic Pitch controller/1P Cyclic Pitch Controller1/M0 Signal Proc./Moving 1P Notch1 ==
  Input : Inport
  GenSpeedIN : Inport  Port=2
  Gain : Gain  Gain=1/Parameters.Turbine.G * rpm2radps(1)
  Moving 2P Filter : cstblocks/Linear Parameter Varying/LPV System  sys=IPCDQ_NF_2P  x0=0  uOffset=0  yOffset=0  xOffset=0  opEquilOption=on  dxOffset=0  sysFixedOption=Use the first model in state-space array  sysFixed=[]  AFixed=false  BFixed=false  CFixed=false  DFixed=false  uDelayFixed=false  yDelayFixed=false  iDelayFixed=false  IMethod=Linear  EMethod=Clip  IndexSearch=Binary search  IndexBegin=on  OutputX=off  OutputXdot=off  OutputLTI=off  OutputOP=off  DataType=double  SimMode=Interpreted execution  InitBufferSize=1024  FixedBuffer=off
  Rate Transition : RateTransition  OutPortSampleTime=DT
  Slow Low Pass for Param : DiscreteStateSpace  A=dLPF_slow.a  B=dLPF_slow.b  C=dLPF_slow.c  D=dLPF_slow.d  SampleTime=DT
  Output : Outport  VectorParamsAs1DForOutWhenUnconnected=off
  wires:
  Moving 2P Filter/1 -> Rate Transition/1
  Slow Low Pass for Param/1 -> Gain/1
  Gain/1 -> Moving 2P Filter/2
  Input/1 -> Moving 2P Filter/1
  GenSpeedIN/1 -> Slow Low Pass for Param/1
  Rate Transition/1 -> Output/1

== system AD_SOAR_c7_V2f_c73_Clean_FullOrderControllerTest/Baseline Controller/Cyclic Pitch controller/1P Cyclic Pitch Controller1/M0 Signal Proc./Moving 2P Notch2 ==
  Input : Inport
  GenSpeedIN : Inport  Port=2
  Gain : Gain  Gain=1/Parameters.Turbine.G * rpm2radps(1) * 2
  Moving 2P Filter : cstblocks/Linear Parameter Varying/LPV System  sys=IPCDQ_NF_2P  x0=0  uOffset=0  yOffset=0  xOffset=0  opEquilOption=on  dxOffset=0  sysFixedOption=Use the first model in state-space array  sysFixed=[]  AFixed=false  BFixed=false  CFixed=false  DFixed=false  uDelayFixed=false  yDelayFixed=false  iDelayFixed=false  IMethod=Linear  EMethod=Clip  IndexSearch=Binary search  IndexBegin=on  OutputX=off  OutputXdot=off  OutputLTI=off  OutputOP=off  DataType=double  SimMode=Interpreted execution  InitBufferSize=1024  FixedBuffer=off
  Rate Transition : RateTransition  OutPortSampleTime=DT
  Slow Low Pass for Param : DiscreteStateSpace  A=dLPF_slow.a  B=dLPF_slow.b  C=dLPF_slow.c  D=dLPF_slow.d  SampleTime=DT
  Output : Outport  VectorParamsAs1DForOutWhenUnconnected=off
  wires:
  Rate Transition/1 -> Output/1
  GenSpeedIN/1 -> Slow Low Pass for Param/1
  Input/1 -> Moving 2P Filter/1
  Gain/1 -> Moving 2P Filter/2
  Slow Low Pass for Param/1 -> Gain/1
  Moving 2P Filter/1 -> Rate Transition/1

== matlab function AD_SOAR_c7_V2f_c73_Clean_FullOrderControllerTest/Baseline Controller/Yaw Controller/Winddirection(deg) ==
  data: Windx input; Windy input; Wdo output
function Wdo  = Wdirection(Windx, Windy)
Wd=atan2(Windx,Windy);
Wdo=Wd+pi/2;

== matlab function AD_SOAR_c7_V2f_c73_Clean_FullOrderControllerTest/Baseline Controller/Wind Speed Estimator/MATLAB Function ==
  data: omega_g input; tau_g input; beta input; WE_params input; A_op input; vh output; xh input; P input; K input; xh output; P output; K output; dt input; Cx parameter; Debug output
function [vh,xh,P,K,Debug] = WSE_EKF(omega_g, tau_g, beta, WE_params, A_op, xh,P,K,dt, Cx)
% This function defines a WSE based off of an Extended Kalman Filter
% Inputs:
% Outputs:
% Nikhar Abbas

% Load R variables
J           = WE_params(1);             % Rotor Inertia
rho         = WE_params(2);             % Air density
Rr          = WE_params(3);             % Rotor Radius, R
Ng          = WE_params(4);             % Gearbox Ratio
ConeAngle   = WE_params(5);                % Cone Angle deg
ShaftTilt   = WE_params(6);                % Shaft Tilt deg

% Constants
H       = [1 0 0];
R       = 0.05;
L       = 4 * Rr;
Ti      = 0.2;

% MANDAR EDIT
% A       = pi*Rr^2;   % Rotor Swept Area, m^2 % ORIGINAL
A       = ( pi * ( Rr*cosd(ConeAngle) )^2 * cosd(ShaftTilt) ); % Projected Rotor Swept Area, m^2

% organize Inputs
om_r    = xh(1);
v_t     = xh(2);
v_m     = xh(3);
om_m    = omega_g  / Ng;

% Find current estimated operating conditions, and saturate
v_r     = v_t + v_m;
% MANDAR EDIT
% lambda  = om_r * Rr / v_r; % ORIGINAL
lambda  = om_r * Rr * cosd(ConeAngle) / v_r;
lambda  = max( min(lambda, Cx.TSR(end)), Cx.TSR(1));


% A_op (system pole) interpolation
% A_op    = interp1(R.WE_FOPoles_v,R.WE_FOPoles,xh(1) + xh(2));


% Cp interpolation
Cp      = interp2(Cx.BlPitch* pi/180, Cx.TSR, Cx.Cpmat, beta, lambda);
Cp      = max(0,Cp);


% Calculate Jacobians
F       = zeros(3,3);

F(1,1)      = A_op;
F(1,2)      = 1/(2*J)*rho*A*Cp*3*(v_m+v_t)^2*1/om_r;
F(1,3)      = 1/(2*J)*rho*A*Cp*3*(v_m+v_t)^2*1/om_r;

F(2,2)      = pi * v_m / (2*L);
F(2,3)      = pi * v_t / (2*L);  % this was 0


% Calculate Covariance
Q           = zeros(3,3);
Q(1,1)      = 1e-5;                     %in DZ WSE, 1e-6
Q(2,2)      = pi * v_m^3 * Ti^2 / L;
Q(3,3)      = 2^2/600;


%% Prediction Update

% states
tau_r       = 1/2 * rho * A * Cp * v_r^3 / om_r;       % Torque calculation
a           = pi * v_m / (2 * L);                           % Wind variance
dom_r       = 1/J * (tau_r - Ng * tau_g);
dv_t        = -a*v_t;
dv_m        = 0;
dxh         = [dom_r; dv_t; dv_m];

% forward euler
xh          = xh + dt*dxh;

% covariance
dP          = F*P + P*F' + Q - K*R*K';
P           = P + dt*dP;

% kalman gain
S           = H*P*H' + R;
K           = P * H' / S(1,1);   %DZ: this is odd, keep an eye on
% K           = P * H' * inv(S);   %DZ: this is odd, keep an eye on...was probably giving NJA stability issues

% output residual & update
y_til       = om_m - om_r;
xh          = xh + K*y_til;
P           = (eye(3) - K * H) * P;         % DZ: this is also different, but I think I've seen this form before


% Output Wind Speed Estimate
vh = v_m + v_t;

% Set Debug Outputs
Debug = Cp;

end

== matlab function AD_SOAR_c7_V2f_c73_Clean_FullOrderControllerTest/Baseline Controller/Yaw Controller/ Yaw Control ==
  data: yawposeCommand output; time input; yawinc input; YAWCW input; YAWCCW input; YAWBRAKEYAW input; YawPos input; Yaw_status input; YawRate input; WINDSPEED input; WindDir input; yawinco output; YAWCWo output; YAWCCWo output; YAWBRAKEYAWo output; Yaw_statuso output; YAWERROR output
function [ yawposeCommand,yawinco,YAWCWo,YAWCCWo,YAWBRAKEYAWo,Yaw_statuso,YAWERROR]= Yaw(time,yawinc ,YAWCW,YAWCCW,YAWBRAKEYAW,YawPos,Yaw_status,YawRate,WINDSPEED, WindDir)
YAWERROR=(WindDir-YawPos*pi/180);
% yawinccheck=Simulation.DT*60000; 
yawinccheck=0.0125;%*60000;
%% Check if are currently yawing
if YAWCW~=0 || YAWCCW~=0    %Yawing already
    
    %%check that we've reached our destination
    if YAWCW && YawPos> yawinc || YAWCCW && YawPos< yawinc
        YAWCWo=0;
        YAWCCWo=0;
        yawinco=0;
        YAWBRAKEYAWo=0;
        yawposeCommand=0; % need to check
        Yaw_statuso=0;
        %YAWERROR_SV=YAWERROR_FV; ????
        %YAWERROR=YAWERROR;%?
        
    else
        YAWCWo=YAWCW;
        YAWCCWo=YAWCCW;
        yawinco=yawinc;%check
        yawposeCommand= yawinc;%YAWERROR+YawPos; % need to check
        YAWBRAKEYAWo=1;% need to check
        Yaw_statuso=1;
        
    end
    
    
    
    
    
%% Check if not currenlty yawing ,accumulate yaw error in  yawinc
 
else

    
    YAWCWo  = YAWCW ;
    YAWCCWo = YAWCCW ;
    yawinco = yawinc ;% need to check
    yawposeCommand = yawinc ; % need to check
    YAWBRAKEYAWo=YAWBRAKEYAW;
    Yaw_statuso = Yaw_status ;   
    
    
    
    
       if  abs(WINDSPEED)>4.0 && Yaw_status==0 && YAWBRAKEYAW == 0
                                                                                           
                if YAWERROR < 0
                    yawinco=yawinc-YAWERROR^2;
%                     YAWCWo=0;
%                     YAWCCWo=0;
%                     YAWBRAKEYAWo=0;
%                     yawposeCommand=yawinc-YAWERROR^2; % need to check
%                     Yaw_statuso=0;
                else
                    yawinco=yawinc+YAWERROR^2;
%                     YAWCWo=0;
%                     YAWCCWo=0;
%                     YAWBRAKEYAWo=0;
%                     yawposeCommand=yawinc-YAWERROR^2; % need to check
%                     Yaw_statuso=0;
                end
      end 
     if  abs( WINDSPEED )<1 && Yaw_status==0 &&YAWBRAKEYAW  == 0
            yawinco = 0;
            YAWCWo=0;
            YAWCCWo=0;
             YAWBRAKEYAWo=0;
            yawposeCommand=0; 
            Yaw_statuso=0;

     end
%         else 
%              
%            yawinco = yawinc; 
%            YAWCWo=YAWCW;
%            YAWCCWo=YAWCCW;
%            YAWBRAKEYAWo=YAWBRAKEYAW;
%            yawposeCommand=yawinc; % need to check
% %            Yaw_statuso=0;
%      end  
      
    
 %%If yawinc exceeds certain limits, decide to start yawing
      
     if yawinc > yawinccheck || yawinc <-1 * yawinccheck  %10 degree error for 10 minutes
%         yawposeCommand = YawPos + yawinc_temp;
        Yaw_statuso =1;
        YAWBRAKEYAWo= 1;
        yawinco=YawPos-YAWERROR;
        YAWCWo=1;
        YAWCCWo=1;
        yawposeCommand=YawPos-YAWERROR; % need to check
                   
%       if (YAWBRAKEPRESS < 500)  %wait until Pressure is under 500 to %       %delay can be used 
%       start yawing 
%       pause(2.0)
%      yawinc=YAWPOS-YAWERROR;


                        if     yawinc <= YawPos %Yaw CCW
                                YAWCWo  = 0 ;
                                YAWCCWo = 1 ;

                            else                 %Yaw CW
                                YAWCWo  = 1;
                                YAWCCWo = 0;
                        end


     end
      
     

    
    
end 
    
 
    
    
%     YAWCWo  = YAWCW ;
%     YAWCCWo = YAWCCW ;
%     yawinco = yawinc ;% need to check
%     yawposeCommand = yawinc ; % need to check
%     Yaw_statuso = Yaw_status ;
    
end

== matlab function AD_SOAR_c7_V2f_c73_Clean_FullOrderControllerTest/Baseline Controller/PID Pitch controller/Variable Saturator1 ==
  data: pitchCommand input; lowerLimit input; pitchCommandOut output; upperLimit input; atLimit output
function [pitchCommandOut,atLimit] = variableSat(pitchCommand,lowerLimit,upperLimit)
%#codegen

if pitchCommand < lowerLimit
    pitchCommandOut = lowerLimit;
    atLimit          = 1;
    
elseif pitchCommand > upperLimit
    pitchCommandOut = upperLimit;
    atLimit         = 1;
    
else
    pitchCommandOut = pitchCommand;
    atLimit         = 0;
end

== matlab function AD_SOAR_c7_V2f_c73_Clean_FullOrderControllerTest/Baseline Controller/Wind Speed Estimator/Soft Start ==
  data: startTime input; out output; endTime input; time input; generic input; actual input
function out = softStart(startTime,endTime,time,generic,actual)

as  = Af_sigma(startTime,endTime);
T   = [time^3,time^2,time,1]';

if time < startTime
    act = 0;
    gen = 1;
elseif time >= startTime && time < endTime
    act = as * T; 
    gen = 1 - as * T;
else
    act = 1;
    gen = 0;
end

out = act*actual + gen*generic;

== matlab function AD_SOAR_c7_V2f_c73_Clean_FullOrderControllerTest/Baseline Controller/Cyclic Pitch controller/1P Cyclic Pitch Controller1/Lead Correction ==
  data: bdq input; b_cos output size=1; psi_o input; b_sin output size=1
function [b_cos,b_sin] = fcn(bdq, psi_o)
% This block supports the Embedded MATLAB subset.
% See the help menu for details. 

b_cos=[cosd(psi_o) sind(psi_o)]*bdq;
b_sin=[-sind(psi_o) cosd(psi_o)]*bdq;

== matlab function AD_SOAR_c7_V2f_c73_Clean_FullOrderControllerTest/Baseline Controller/Cyclic Pitch controller/1P Cyclic Pitch Controller1/d-q transformation ==
  data: RootMyb input; M_d output; Az input; M_q output; NumBl input
function [M_d,M_q] = fwdMBC2(RootMyb, Az, NumBl)
% This block supports the Embedded MATLAB subset.
% See the help menu for details.

if NumBl == 2
    
    My=RootMyb-mean(RootMyb(1:2)); %remove mean
    
    M_d = [cosd(Az) cosd(Az+180) 0]*My;
    M_q =  [sind(Az) sind(Az+180) 0]*My;
else
%     My=RootMyb-mean(RootMyb); %remove mean
    My=RootMyb;
    M_d = (2/3).*[cosd(Az) cosd(Az+120) cosd(Az+240)]*My;
    M_q =  (2/3).*[sind(Az) sind(Az+120) sind(Az+240)]*My;
end

== matlab function AD_SOAR_c7_V2f_c73_Clean_FullOrderControllerTest/Baseline Controller/Cyclic Pitch controller/1P Cyclic Pitch Controller1/inverse d-q transformation ==
  data: bdq input; b1 output size=1; Az input; b2 output size=1; NumBl input; b3 output size=1
function [b1,b2,b3] = bckMBC2(bdq, Az, NumBl)
% This block supports the Embedded MATLAB subset.
% See the help menu for details.


if NumBl == 2
    
    b1=[cosd(Az) sind(Az)]*bdq;
    b2=[cosd(Az - 180) sind(Az - 180)]*bdq;
    b3=0;
    
else
    b1=[cosd(Az) sind(Az)]*bdq;
    b2=[cosd(Az + 120) sind(Az + 120)]*bdq;
    b3=[cosd(Az + 240) sind(Az + 240)]*bdq;
    
end

== matlab function AD_SOAR_c7_V2f_c73_Clean_FullOrderControllerTest/Baseline Controller/Cyclic Pitch controller/1P Cyclic Pitch Controller1/saturation (limit schedule)1 ==
  data: bdq_unsat input size=[2 1]; bdq output; b_avg input; M0 input; PitchControlParams parameter; k output
%limit b_d and b_q so b_1,2,or3 does not get bigger than b_avg (the sinusoids don't get cut off at zero)
%unless b_avg is <0, then limit to 0
%at_limit is 1 if limited, 0 otherwise

function [bdq,k]  = fcn(bdq_unsat, b_avg, M0,PitchControlParams)

MODE    = PitchControlParams.IPCDQ_MODE;  % 1 no IPC below rated (no power loss), 2 IPC always on, 3
M0_set  = PitchControlParams.IPCDQ_M0_set;
k_sat   = PitchControlParams.IPCDQ_k_sat;

if MODE == 1
    
    if (b_avg <=deg2rad(PitchControlParams.theta_fine + 1))
        bdq=[0;0];
        k = 0;
    else
        if (norm(bdq_unsat,2) <= b_avg)
            bdq = bdq_unsat;
            k = 1;
        else
            bdq=bdq_unsat*(b_avg/norm(bdq_unsat,2));
            k = (b_avg/norm(bdq_unsat,2));
        end
    end
elseif MODE == 2
    %     if (b_avg <= deg2rad(PitchControlParams.theta_fine+0.05))
    %         bdq=[0;0];
    %         k = 0;
    %     else
    if (norm(bdq_unsat,2) > deg2rad(15))
        bdq = bdq_unsat*(deg2rad(15)/norm(bdq_unsat,2));
        k = (deg2rad(15)/norm(bdq_unsat,2));
    else
        bdq = bdq_unsat;
        k = 1;
    end
    %     end
else  % MODE 3
    if (M0 > M0_set - 1/(2*k_sat))
        if (M0 > M0_set + 1/(2*k_sat))
            bdq = bdq_unsat;
            k = 1;
        else
            k = k_sat*(M0-M0_set)+1/2;
            bdq = k*bdq_unsat;
        end
    else
        bdq = [0;0];
        k = 0;
    end
end
%
% if (b_avg <=0)
%         bdq = bdq_unsat;
% else
%     if (norm(bdq_unsat,2) <= b_avg)
%         bdq = bdq_unsat;
%     else
%         bdq = bdq_unsat;
%     end
% end

== matlab function AD_SOAR_c7_V2f_c73_Clean_FullOrderControllerTest/Baseline Controller/Torque Controller/LUT-Based Torque Control/Baseline Torque Cotnroller ==
  settings: updateMethod=DISCRETE  sampleTime=Control.DT
  data: W_hss input; Pitch input; genTorque output; region output; S_LowBPLim input; TorqueControlParams parameter
function [genTorque, region] = regionSelectTq_Flex( W_hss, Pitch, S_LowBPLim, TorqueControlParams)
% This block supports an embeddable subset of the MATLAB language.
% See the help menu for details.


%% Assign Constants

wg_rated    = TorqueControlParams.wg_rated;
T_rated     = TorqueControlParams.T_rated;
w2_high     = TorqueControlParams.w2_high;
w1_high     = TorqueControlParams.w1_high;
wg_min      = TorqueControlParams.wg_min;
m2_5        = TorqueControlParams.m2_5;
c2_5        = TorqueControlParams.c2_5;
m1_5        = TorqueControlParams.m1_5;
c1_5        = TorqueControlParams.c1_5;
k_opt       = TorqueControlParams.k_opt;


%% Switch based on Gen. Speed

if (((S_LowBPLim==0)&&(W_hss >= wg_rated)) || ((S_LowBPLim==1)&&((Pitch >= TorqueControlParams.fine_pitch+3) || (W_hss >= wg_rated)))) %Region 3 calcs
    region=3;
    genTorque = T_rated;

elseif (W_hss >= w2_high)                %Region 2.5
    region=2.5;    
%     genTorque = m2_5 * W_hss + c2_5;
    genTorque = k_opt * W_hss^2; % MANDAR TEST
elseif (W_hss >= w1_high)                    %Region 2
    region=2;
    genTorque = k_opt * W_hss^2;
    
elseif (W_hss > wg_min)                    %Region 1.5
    region=1.5;
        genTorque = m1_5 * W_hss + c1_5;
%     genTorque = k_opt * W_hss^2; % MANDAR TEST
else                                    %Region 1
    region=1;
    genTorque = 0;
end

% if startup
%     region=1;
%     genTorque = 0;
% end
